simulink model "lorenzSystem"  (R2020b)
settings: Solver=VariableStepAuto  StartTime=0.0  StopTime=60  RelTol=1e-8
values from neighbouring files (symbols this model uses):
  b = 8/3    (= 2.66666666667)    [aae666_hw1_ex9.m]
  r = 28    [aae666_hw1_ex9.m]
  sigma = 10    [aae666_hw1_ex9.m]
  x1_0 = 0    [aae666_hw1_ex9.m]
  x2_0 = 1+eps    [aae666_hw1_ex9.m]
  x3_0 = 0    [aae666_hw1_ex9.m]
settings Model: Creator=Tomo  LastModifiedBy=Tomo

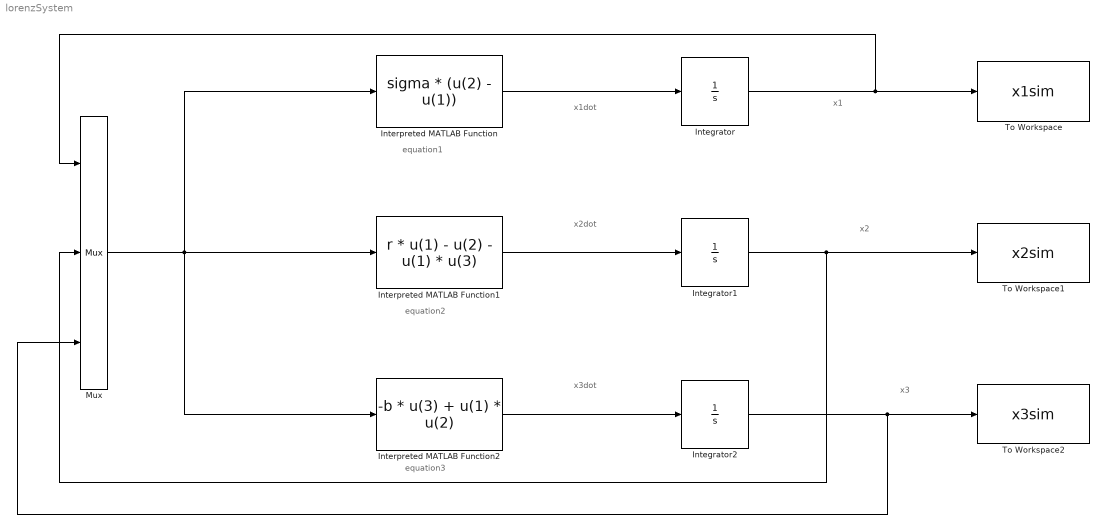
== system lorenzSystem ==
  note: equation1
  note: x1
  note: x2
  note: x3
  note: x1dot
  note: x2dot
  note: x3dot
  note: equation2
  note: equation3
  Integrator : Integrator  InitialCondition=x1_0
  Integrator1 : Integrator  InitialCondition=x2_0
  Integrator2 : Integrator  InitialCondition=x3_0
  Interpreted MATLAB Function : MATLABFcn  MATLABFcn=sigma * (u(2) - u(1))
  Interpreted MATLAB Function1 : MATLABFcn  MATLABFcn=r * u(1) - u(2) - u(1) * u(3)
  Interpreted MATLAB Function2 : MATLABFcn  MATLABFcn=-b * u(3) + u(1) * u(2)
  Mux : Mux  Inputs=3
  To Workspace : ToWorkspace  VariableName=x1sim  SaveFormat=Structure With Time  SampleTime=-1
  To Workspace1 : ToWorkspace  VariableName=x2sim  SaveFormat=Structure With Time  SampleTime=-1
  To Workspace2 : ToWorkspace  VariableName=x3sim  SaveFormat=Structure With Time  SampleTime=-1
  wires:
  Integrator/1 -> Mux/1, To Workspace/1
  Integrator1/1 -> Mux/2, To Workspace1/1
  Integrator2/1 -> Mux/3, To Workspace2/1
  Mux/1 -> Interpreted MATLAB Function/1, Interpreted MATLAB Function2/1, Interpreted MATLAB Function1/1
  Interpreted MATLAB Function/1 -> Integrator/1
  Interpreted MATLAB Function1/1 -> Integrator1/1
  Interpreted MATLAB Function2/1 -> Integrator2/1
